simulink model "Quadrotor_Model_PID_Control"  (R2023b)
settings: Solver=VariableStepAuto  StartTime=0.0  StopTime=10.0  RelTol=1e-3
values from neighbouring files (symbols this model uses):
  b = 1.140 * 10^-7    (= 1.14e-07)    [Quadrotor_PID_Parameter_Trial_Updated.m]
  g = 9.82    [Quadrotor_PID_Parameter_Trial_Updated.m]
  I_xx = 4.856 * 10^-3    (= 0.004856)    [Quadrotor_PID_Parameter_Trial_Updated.m]
  I_yy = 4.856 * 10^-3    (= 0.004856)    [Quadrotor_PID_Parameter_Trial_Updated.m]
  I_zz = 8.801 * 10^-3    (= 0.008801)    [Quadrotor_PID_Parameter_Trial_Updated.m]
  k = 2.980*10^-6    (= 2.98e-06)    [Quadrotor_PID_Parameter_Trial_Updated.m]
  Kdx = 1.5    [Quadrotor_PID_Parameter_Trial_Updated.m]
  Kdy = 2.5    [Quadrotor_PID_Parameter_Trial_Updated.m]
  Kdz = 1    [Quadrotor_PID_Parameter_Trial_Updated.m]
  l = 0.225    [Quadrotor_PID_Parameter_Trial_Updated.m]    (also in Reference_Drone_Updated_PID.m = 0.15)
  m = 0.468    [Quadrotor_PID_Parameter_Trial_Updated.m]
libraries: slpidlib x4
settings Model: Creator=jerss  LastModifiedBy=jerss

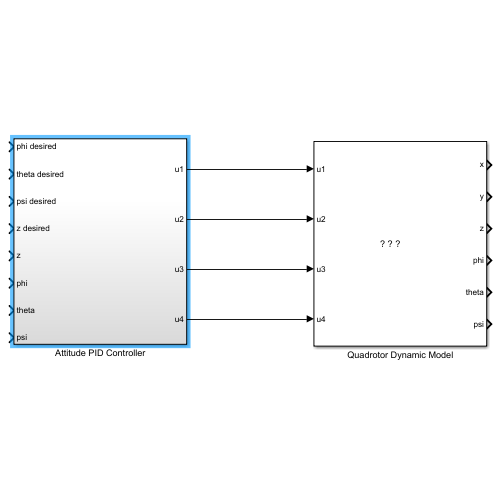
[thumbnail: Simulink's stored preview of the top-level diagram]
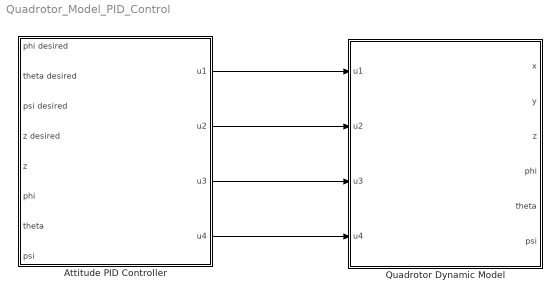
== system Quadrotor_Model_PID_Control ==
  Attitude PID Controller : Subsystem
  Quadrotor Dynamic Model : Subsystem
      mask Display: image('C:\Users\angel\OneDrive - Universidad Politécnica de Yucatán\CIMAT\1st semester\Robotic Systems Modeling and Control\Project\Quadrotor\images\quadrotor.jpg');
  wires:
  Attitude PID Controller/1(u1) -> Quadrotor Dynamic Model/1(u1)
  Attitude PID Controller/2(u2) -> Quadrotor Dynamic Model/2(u2)
  Attitude PID Controller/3(u3) -> Quadrotor Dynamic Model/3(u3)
  Attitude PID Controller/4(u4) -> Quadrotor Dynamic Model/4(u4)

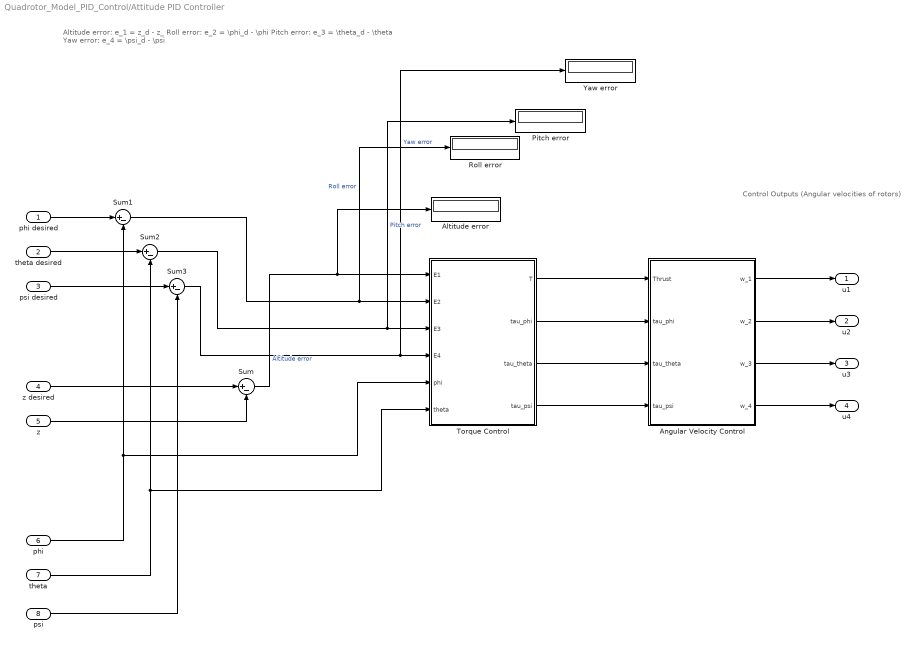
== system Quadrotor_Model_PID_Control/Attitude PID Controller ==
  note: Control Outputs
      | (Angular velocities of rotors)
  note: Altitude error: e_1 = z_d - z_
      | Roll error: e_2 = \phi_d - \phi
      | Pitch error: e_3 = \theta_d - \theta
      | Yaw error: e_4 = \psi_d - \psi
  phi desired : Inport
  theta desired : Inport  Port=2
  psi desired : Inport  Port=3
  z desired : Inport  Port=4
  z : Inport  Port=5
  phi : Inport  Port=6
  theta : Inport  Port=7
  psi : Inport  Port=8
  Altitude error : Display
  Angular Velocity Control : Subsystem
  Pitch error : Display
  Roll error : Display
  Sum{,1..3} (4 alike) : Sum  Inputs=|+-
  Torque Control : Subsystem
  Yaw error : Display
  u1 : Outport
  u2 : Outport  Port=2
  u3 : Outport  Port=3
  u4 : Outport  Port=4
  wires:
  z desired/1 -> Sum/1
  z/1 -> Sum/2
  Sum/1 -> Altitude error/1, Torque Control/1(E1)  "Altitude error"
  phi desired/1 -> Sum1/1
  phi/1 -> Torque Control/5("phi "), Sum1/2
  theta desired/1 -> Sum2/1
  theta/1 -> Sum2/2, Torque Control/6("theta ")
  psi desired/1 -> Sum3/1
  psi/1 -> Sum3/2
  Sum1/1 -> Roll error/1, Torque Control/2(E2)  "Roll error"
  Sum2/1 -> Pitch error/1, Torque Control/3(E3)  "Pitch error"
  Sum3/1 -> Torque Control/4(E4), Yaw error/1  "Yaw error"
  Torque Control/2(tau_phi) -> Angular Velocity Control/2(tau_phi)
  Torque Control/1(T) -> Angular Velocity Control/1(Thrust)
  Torque Control/3(tau_theta) -> Angular Velocity Control/3(tau_theta)
  Torque Control/4(tau_psi) -> Angular Velocity Control/4("tau_psi ")
  Angular Velocity Control/1(w_1) -> u1/1
  Angular Velocity Control/2(w_2) -> u2/1
  Angular Velocity Control/3(w_3) -> u3/1
  Angular Velocity Control/4("w_4 ") -> u4/1

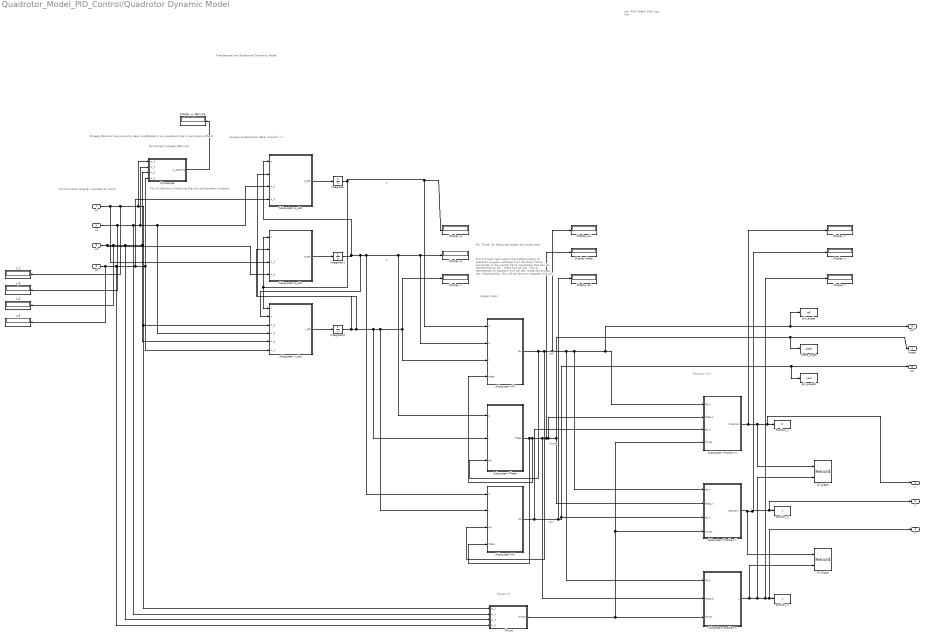
== system Quadrotor_Model_PID_Control/Quadrotor Dynamic Model ==
  note: Phi, Theta, Psi Measured angles dot inside here
  note: This W_Gamma is following the plus configuration currently
  note: Omega_Gamma have currently been unreflected in our equations due to gyroscopic effects
  note: This full block talks about the trabsformation of quadrotor angular velocities from the body frame coordinate to the inertial frame coordinate that can be represented by phi , theta and psi dot - this is represented by equation 6 of phi dot, theta dot and psi dot.
      | Subsequently, this will be done to integrate it to phi, theta and psi.
  note: Angular Accelerations (Body Frame) (\nu)
  note: .
  note: \phi: Roll
      | \theta: Pitch
      | \psi: Yaw
  note: Control Inputs
      | (Angular velocities of rotors)
  note: Positions (\xi)
  note: Angles (\eta)
  note: Gyroscope (\omega_\Gamma)
  note: Thrust (T)
  note: p
  note: q
  note: r
  note: \phi
  note: \theta
  note: \psi
  note: Translational and Rotational Dynamics Model
  u1 : Inport
  u2 : Inport  Port=2
  u3 : Inport  Port=3
  u4 : Inport  Port=4
  Display p : Display
  Display phi : Display
  Display psi : Display
  Display q : Display
  Display r : Display
  Display theta : Display
  Display w_Gamma : Display
  Display x : Display
  Display y : Display
  Display z : Display
  Gyroscope : MATLAB Function  TreatAsAtomicUnit=on
  Integrator : Integrator
  Integrator1 : Integrator
  Integrator2 : Integrator
  Position_x : ToWorkspace  VariableName=X  SampleTime=-1
  Subsystem Phi : Subsystem
  Subsystem Position X : Subsystem
  Subsystem Position Y : Subsystem
  Subsystem Psi : Subsystem
  Subsystem Theta : Subsystem
  Subsystem p_dot : Subsystem
  Subsystem position z : Subsystem
  Subsystem q_dot : Subsystem
  Subsystem r_dot : Subsystem
  Thrust : MATLAB Function  TreatAsAtomicUnit=on
  XZ graph : Record  FileSettingsInternal="{\"entries\":[{\"content\":{\"excelSettings\":{\"content\":{},\"type\":\"Streamout.ExcelSettings\"}},\"type\":\"Streamout.FileSettingStorage\",\"uuid\":\"\"}],\"packageUris\":[\"http:\\/\\/schema.mathworks.com\\/mf0\\/streamout_blocks\\/R2020a\"],\"version\":\"1.0\"}"  Layout=[1 1]  SignalsInternal="{\"entries\":[{\"content\":{\"signals\":[{\"content\":{\"blockPath\":[],\"dimensions\":[1],\"domain\":\"\",\"lineColor\":\"#a2142f\",\"plots\":[1],\"port\":1,\"signalID\":16,\"signalName\":\"Subsystem position x\"},\"type\":\"RecordBlkView.Signal\",\"uuid\":\"\"},{\"content\":{\"blockPath\":[],\"dimensions\":[1],\"domain\":\"\",\"lineColor\":\"#139fff\",\"plots\":[1],\"port\":2,\"signalID\":19,\"signalName\":\"Subsystem position z\"},\"type\":\"RecordBlkView.Signal\",\"uuid\":\"\"}]},\"type\":\"RecordBlkView.InputSignals\",\"uuid\":\"\"}],\"packageUris\":[\"http:\\/\\/schema.mathworks.com\\/mf0\\/streamout_blocks\\/R2020a\"],\"version\":\"1.0\"}"  VisualizationBindings="{\"xyplotplugin\":{\"info\":[{\"series\":[{\"bindingParametersList\":[{\"parameter\":\"X-Axis\",\"signalID\":16,\"signalName\":\"Subsystem position x\"},{\"parameter\":\"Y-Axis\",\"signalID\":19,\"signalName\":\"Subsystem position z\"}],\"seriesID\":56291}],\"subplotID\":1}]}}"  CompatibilityTag=XY  st=-1
  YZ Graph : Record  FileSettingsInternal="{\"entries\":[{\"content\":{\"excelSettings\":{\"content\":{},\"type\":\"Streamout.ExcelSettings\"}},\"type\":\"Streamout.FileSettingStorage\",\"uuid\":\"\"}],\"packageUris\":[\"http:\\/\\/schema.mathworks.com\\/mf0\\/streamout_blocks\\/R2020a\"],\"version\":\"1.0\"}"  Layout=[1 1]  SignalsInternal="{\"entries\":[{\"content\":{\"signals\":[{\"content\":{\"blockPath\":[],\"dimensions\":[1],\"domain\":\"\",\"lineColor\":\"#a2142f\",\"plots\":[1],\"port\":1,\"signalID\":8,\"signalName\":\"Subsystem position y\"},\"type\":\"RecordBlkView.Signal\",\"uuid\":\"\"},{\"content\":{\"blockPath\":[],\"dimensions\":[1],\"domain\":\"\",\"lineColor\":\"#139fff\",\"plots\":[1],\"port\":2,\"signalID\":11,\"signalName\":\"Subsystem position z\"},\"type\":\"RecordBlkView.Signal\",\"uuid\":\"\"}]},\"type\":\"RecordBlkView.InputSignals\",\"uuid\":\"\"}],\"packageUris\":[\"http:\\/\\/schema.mathworks.com\\/mf0\\/streamout_blocks\\/R2020a\"],\"version\":\"1.0\"}"  VisualizationBindings="{\"xyplotplugin\":{\"info\":[{\"series\":[{\"bindingParametersList\":[{\"parameter\":\"X-Axis\",\"signalID\":8,\"signalName\":\"Subsystem position y\"},{\"parameter\":\"Y-Axis\",\"signalID\":11,\"signalName\":\"Subsystem position z\"}],\"seriesID\":24584}],\"subplotID\":1}]}}"  CompatibilityTag=XY  st=-1
  phi_angle : ToWorkspace  VariableName=roll  SampleTime=-1
  phi_angle1 : ToWorkspace  VariableName=yaw  SampleTime=-1
  position_y : ToWorkspace  VariableName=y  SampleTime=-1
  position_z : ToWorkspace  VariableName=z  SampleTime=-1
  theta_angle : ToWorkspace  VariableName=pitch  SampleTime=-1
  u_{1..4} (4 alike) : Display
  x : Outport
  y : Outport  Port=2
  z : Outport  Port=3
  phi : Outport  Port=4
  theta : Outport  Port=5
  psi : Outport  Port=6
  wires:
  u1/1 -> Subsystem q_dot/3(w_1), u_1/1, Gyroscope/1(w_1), Subsystem r_dot/3(w_1), Thrust/1(w_1)
  u2/1 -> Subsystem p_dot/3(w_2), Subsystem r_dot/4(w_2), Gyroscope/2(w_2), Thrust/2(w_2), u_2/1
  u3/1 -> Subsystem q_dot/4(w_3), Gyroscope/3(w_3), Subsystem r_dot/5(w_3), Thrust/3(w_3), u_3/1
  u4/1 -> u_4/1, Gyroscope/4(w_4), Subsystem r_dot/6(w_4), Subsystem p_dot/4(w_4), Thrust/4(w_4)
  Thrust/1(Thrust) -> Subsystem Position X/4(Thrust), Subsystem Position Y/4("Thrust "), Subsystem position z/3(Thrust)
  Subsystem Phi/1("Phi ") -> Subsystem Theta/3("phi "), Subsystem Psi/3(Phi), Display phi/1, Subsystem position z/1("Phi Z "), Subsystem Position Y/1("Phi Y "), phi/1, phi_angle/1, Subsystem Position X/1("Phi X ")
  Subsystem Psi/1(Psi) -> Subsystem Position X/3("Psi X "), Display psi/1, phi_angle1/1, psi/1, Subsystem Position Y/3("Psi Y ")
  Subsystem Position X/1(X Position) -> Display x/1, x/1, Position_x/1, XZ graph/1
  Subsystem position z/1(z) -> YZ Graph/2, XZ graph/2, z/1, position_z/1, Display z/1
  Subsystem Position Y/1("Position Y ") -> y/1, position_y/1, Display y/1, YZ Graph/1
  Gyroscope/1(w_Gamma) -> Display w_Gamma/1
  Subsystem p_dot/1(p_dot) -> Integrator/1
  Subsystem q_dot/1(q_dot) -> Integrator1/1
  Subsystem r_dot/1(r_dot) -> Integrator2/1
  Integrator/1 -> Display p/1, Subsystem Phi/1(p), Subsystem r_dot/1("p "), Subsystem q_dot/1("p ")
  Integrator2/1 -> Subsystem Theta/2(r), Subsystem Psi/2(r), Display r/1, Subsystem Phi/3(r), Subsystem p_dot/2(r), Subsystem q_dot/2(r)
  Integrator1/1 -> Subsystem p_dot/1(q), Subsystem Psi/1(q), Subsystem Theta/1(q), Display q/1, Subsystem Phi/2(q), Subsystem r_dot/2(q)
  Subsystem Theta/1(Theta) -> Subsystem Psi/4(Theta), Subsystem Phi/4(theta), Subsystem position z/2("Theta Z "), Display theta/1, Subsystem Position X/2("Theta X "), theta_angle/1, theta/1, Subsystem Position Y/2("Theta Y ")

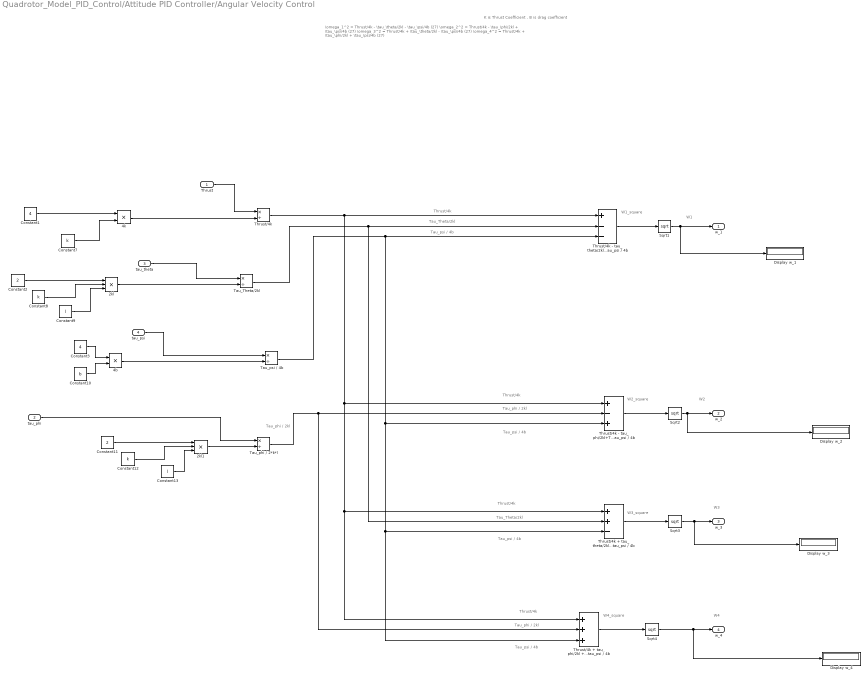
== system Quadrotor_Model_PID_Control/Attitude PID Controller/Angular Velocity Control ==
  note: Tau_psi / 4b
  note: Tau_Theta/2kl
  note: Thrust/4k
  note: W1_square
  note: K is Thrust Coefficient , B is drag coefficient
  note: \omega_1^2 = Thrust/4k - \tau_\theta/2kl - \tau_\psi/4b   (27)
      |
      | \omega_2^2 = Thrust/4k - \tau_\phi/2kl + \tau_\psi/4b   (27)
      |
      | \omega_3^2 = Thrust/4k + \tau_\theta/2kl - \tau_\psi/4b   (27)
      |
      | \omega_4^2 = Thrust/4k + \tau_\phi/2kl + \tau_\psi/4b   (27)
  note: W1
  note: Thrust/4k
  note: Tau_phi / 2kl
  note: Tau_psi / 4b
  note: W2_square
  note: W2
  note: Thrust/4k
  note: W3
  note: W3_square
  note: Tau_Theta/2kl
  note: Tau_psi / 4b
  note: W4_square
  note: W4
  note: Thrust/4k
  note: Tau_phi / 2kl
  note: Tau_phi / 2kl
  note: Tau_psi / 4b
  Thrust : Inport
  tau_phi : Inport  Port=2
  tau_theta : Inport  Port=3
  "tau_psi " : Inport  Port=4
  2kl : Product  Inputs=***
  2kl1 : Product  Inputs=***
  4b : Product  Inputs=**
  4k : Product  Inputs=**
  Constant1 : Constant  Value=4
  Constant10 : Constant  Value=b
  Constant11 : Constant  Value=2
  Constant12 : Constant  Value=k
  Constant13 : Constant  Value=l
  Constant2 : Constant  Value=2
  Constant3 : Constant  Value=4
  Constant7 : Constant  Value=k
  Constant8 : Constant  Value=k
  Constant9 : Constant  Value=l
  Display w_{1..4} (4 alike) : Display
  Sqrt1 : Sqrt
  Sqrt2 : Sqrt  OutputSignalType=real
  Sqrt3 : Sqrt
  Sqrt4 : Sqrt
  Tau_Theta/2kl : Product  Inputs=*/
  Tau_phi / 2*k*l : Product  Inputs=*/
  Tau_psi / 4b : Product  Inputs=*/
  Thrust/4k : Product  Inputs=*/
  Thrust/4k + tau_phi/2kl + tau_psi / 4b : Sum  Inputs=+++
  Thrust/4k + tau_theta/2kl -tau_psi / 4b : Sum  Inputs=++-
  Thrust/4k - tau_phi/2kl+Tau_psi / 4b : Sum  Inputs=+-+
  Thrust/4k - tau_theta/2kl-Tau_psi / 4b : Sum  Inputs=+--
  w_1 : Outport
  w_2 : Outport  Port=2
  w_3 : Outport  Port=3
  "w_4 " : Outport  Port=4
  wires:
  tau_theta/1 -> Tau_Theta/2kl/1
  Sqrt1/1 -> Display w_1/1, w_1/1
  tau_phi/1 -> Tau_phi / 2*k*l/1
  "tau_psi "/1 -> Tau_psi / 4b/1
  Sqrt2/1 -> Display w_2/1, w_2/1
  Thrust/4k - tau_phi/2kl+Tau_psi / 4b/1 -> Sqrt2/1
  Thrust/4k + tau_theta/2kl -tau_psi / 4b/1 -> Sqrt3/1
  Sqrt3/1 -> Display w_3/1, w_3/1
  Thrust/4k + tau_phi/2kl + tau_psi / 4b/1 -> Sqrt4/1
  Sqrt4/1 -> Display w_4/1, "w_4 "/1
  Constant1/1 -> 4k/1
  Constant7/1 -> 4k/2
  Constant8/1 -> 2kl/2
  Constant2/1 -> 2kl/1
  2kl/1 -> Tau_Theta/2kl/2
  Constant9/1 -> 2kl/3
  Constant3/1 -> 4b/1
  Constant10/1 -> 4b/2
  4k/1 -> Thrust/4k/2
  Constant11/1 -> 2kl1/1
  Constant12/1 -> 2kl1/2
  Constant13/1 -> 2kl1/3
  Thrust/1 -> Thrust/4k/1
  4b/1 -> Tau_psi / 4b/2
  2kl1/1 -> Tau_phi / 2*k*l/2
  Thrust/4k/1 -> Thrust/4k + tau_theta/2kl -tau_psi / 4b/1, Thrust/4k + tau_phi/2kl + tau_psi / 4b/1, Thrust/4k - tau_phi/2kl+Tau_psi / 4b/1, Thrust/4k - tau_theta/2kl-Tau_psi / 4b/1
  Tau_Theta/2kl/1 -> Thrust/4k - tau_theta/2kl-Tau_psi / 4b/2, Thrust/4k + tau_theta/2kl -tau_psi / 4b/2
  Thrust/4k - tau_theta/2kl-Tau_psi / 4b/1 -> Sqrt1/1
  Tau_phi / 2*k*l/1 -> Thrust/4k + tau_phi/2kl + tau_psi / 4b/2, Thrust/4k - tau_phi/2kl+Tau_psi / 4b/2
  Tau_psi / 4b/1 -> Thrust/4k - tau_theta/2kl-Tau_psi / 4b/3, Thrust/4k - tau_phi/2kl+Tau_psi / 4b/3, Thrust/4k + tau_phi/2kl + tau_psi / 4b/3, Thrust/4k + tau_theta/2kl -tau_psi / 4b/3

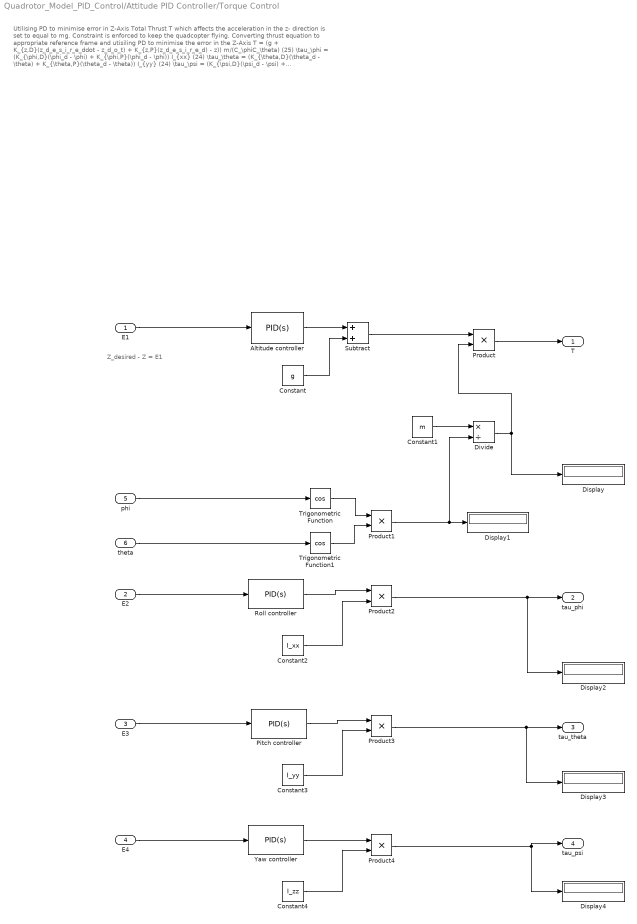
== system Quadrotor_Model_PID_Control/Attitude PID Controller/Torque Control ==
  note: Z_desired - Z = E1
  note: Utilising PD to minimise error in Z-Axis
      | Total Thrust T which affects the acceleration in the z- direction is set to equal to mg.
      | Constraint is enforced to keep the quadcopter flying.
      | Converting thrust equation to appropriate reference frame and utisiling PD to minimise the error in the Z-Axis
      |
      | T = (g + K_{z,D}(z_d_e_s_i_r_e_ddot - z_d_o_t) + K_{z,P}(z_d_e_s_i_r_e_d) - z)) m/(C_\phiC_\theta)     (25)
      |
      | \tau_\phi = (K_{\phi,D}(\phi_d - \phi) + K_{\phi,P}(\phi_d - \phi)) I_{xx}                   (24)
      |
      | \tau_\theta = (K_{\theta,D}(\theta_d - \theta) + K_{\theta,P}(\theta_d - \theta)) I_{yy}                    (24)
      |
      | \tau_\psi = (K_{\psi,D}(\psi_d - \psi) + K_{\psi,P}(\psi_d - \psi)) I_{zz}                (24)
  E1 : Inport
  E2 : Inport  Port=2
  E3 : Inport  Port=3
  E4 : Inport  Port=4
  "phi " : Inport  Port=5
  "theta " : Inport  Port=6
  Altitude controller : slpidlib/PID Controller  Controller=PID  Form=Parallel  TimeDomain=Continuous-time  UseExternalTs=off  SampleTime=-1  IntegratorMethod=Forward Euler  FilterMethod=Forward Euler  ControllerParametersSource=internal  P=57  I=0.001  UseKiTs=off  D=23  N=572.770791824146  UseFilter=on  TunerSelectOption=Transfer Function Based (PID Tuner App)  InitialConditionSource=internal  InitialConditionForIntegrator=0  InitialConditionForFilter=0  DifferentiatorICPrevScaledInput=0  ExternalReset=none  TrackingMode=off  Kt=1  LimitOutput=on  SatLimitsSource=internal  UpperSaturationLimit=5  LowerSaturationLimit=-5  LinearizeAsGain=on  AntiWindupMode=none  Kb=1  LimitIntegrator=off  UpperIntegratorSaturationLimit=inf  LowerIntegratorSaturationLimit=-inf  POutMin=[]  POutMax=[]  IOutMin=[]  IOutMax=[]  DOutMin=[]  DOutMax=[]  NOutMin=[]  NOutMax=[]  SumOutMin=[]  SumOutMax=[]  SaturationOutMin=[]  SaturationOutMax=[]  PParamMin=[]  PParamMax=[]  IParamMin=[]  IParamMax=[]  DParamMin=[]  DParamMax=[]  NParamMin=[]  NParamMax=[]  KbParamMin=[]  KbParamMax=[]  KtParamMin=[]  KtParamMax=[]  KbOutMin=[]  KbOutMax=[]  KtOutMin=[]  KtOutMax=[]  IntegratorOutMin=[]  IntegratorOutMax=[]  FilterOutMin=[]  FilterOutMax=[]  SumI1OutMin=[]  SumI1OutMax=[]  SumI2OutMin=[]  SumI2OutMax=[]  SumI3OutMin=[]  SumI3OutMax=[]  SumI4OutMin=[]  SumI4OutMax=[]  SumDOutMin=[]  SumDOutMax=[]  DifferentiatorOutMin=[]  DifferentiatorOutMax=[]  FilterDiffOutCoefMin=[]  FilterDiffOutCoefMax=[]  ReciprocalOutMin=[]  ReciprocalOutMax=[]  SumDenOutMin=[]  SumDenOutMax=[]  SumNumOutMin=[]  SumNumOutMax=[]  DivideOutMin=[]  DivideOutMax=[]  UdiffTsProdOutMin=[]  UdiffTsProdOutMax=[]  NTsProdOutMin=[]  NTsProdOutMax=[]  UintegralTsProdOutMin=[]  UintegralTsProdOutMax=[]  UngainTsProdOutMin=[]  UngainTsProdOutMax=[]  ClampingZeroOutDataTypeStr=Inherit: Inherit via back propagation  ClampingZeroOutMin=[]  ClampingZeroOutMax=[]  FilterDenConstantOutDataTypeStr=Inherit: Inherit via back propagation  FilterDenConstantOutMin=[]  FilterDenConstantOutMax=[]  PCopyOutDataTypeStr=Inherit: Inherit via back propagation  PCopyOutMin=[]  PCopyOutMax=[]  NCopyOutDataTypeStr=Inherit: Inherit via back propagation  NCopyOutMin=[]  NCopyOutMax=[]  IntegratorContinuousStateAttributes=''  IntegratorStateMustResolveToSignalObject=off  IntegratorRTWStateStorageClass=Auto  FilterContinuousStateAttributes=''  FilterStateMustResolveToSignalObject=off  FilterRTWStateStorageClass=Auto  ParallelPVariant=InternalParameters  IdealPVariant=Disabled  IVariant=InternalParameters  DVariant=InternalParameters  IntegratorVariant=Continuous  SatVariant=Enabled  AWVariant=Passthrough  PCopyVariant=Disabled  TRVariant=Disabled  FdbkBlocksVariant=Forward  IdealPFdbkVariant=Disabled  SatFdbkVariant=Disabled  DerivativeFilterVariant=ContFilter  NVariant=InternalParameters  NCopyVariant=Disabled  FilterICVariant=InternalICsFilter  IntegratorICVariant=InternalICs  ExternalResetVariant=Disabled  TRSumVariant=Passthrough  SumFdbkVariant=Disabled  SumVariant=Sum_PID  TsampFilterVariant=InternalTs  TsampNgainVariant=Passthrough  TsampIntegralVariant=Disabled_SignalSpec  ExternalSaturationOutDataTypeStr=Inherit: Same as second input
  Constant : Constant  Value=g
  Constant1 : Constant  Value=m
  Constant2 : Constant  Value=I_xx
  Constant3 : Constant  Value=I_yy
  Constant4 : Constant  Value=I_zz
  Display{,1..4} (5 alike) : Display
  Divide : Product  Inputs=*/
  Pitch controller : slpidlib/PID Controller  Controller=PID  Form=Parallel  TimeDomain=Continuous-time  UseExternalTs=off  SampleTime=-1  IntegratorMethod=Forward Euler  FilterMethod=Forward Euler  ControllerParametersSource=internal  P=55  I=0.01  UseKiTs=off  D=11  N=1414.64809761679  UseFilter=on  TunerSelectOption=Transfer Function Based (PID Tuner App)  InitialConditionSource=internal  InitialConditionForIntegrator=0  InitialConditionForFilter=0  DifferentiatorICPrevScaledInput=0  ExternalReset=none  TrackingMode=off  Kt=1  LimitOutput=on  SatLimitsSource=internal  UpperSaturationLimit=0.9  LowerSaturationLimit=-0.9  LinearizeAsGain=on  AntiWindupMode=none  Kb=1  LimitIntegrator=off  UpperIntegratorSaturationLimit=inf  LowerIntegratorSaturationLimit=-inf  POutMin=[]  POutMax=[]  IOutMin=[]  IOutMax=[]  DOutMin=[]  DOutMax=[]  NOutMin=[]  NOutMax=[]  SumOutMin=[]  SumOutMax=[]  SaturationOutMin=[]  SaturationOutMax=[]  PParamMin=[]  PParamMax=[]  IParamMin=[]  IParamMax=[]  DParamMin=[]  DParamMax=[]  NParamMin=[]  NParamMax=[]  KbParamMin=[]  KbParamMax=[]  KtParamMin=[]  KtParamMax=[]  KbOutMin=[]  KbOutMax=[]  KtOutMin=[]  KtOutMax=[]  IntegratorOutMin=[]  IntegratorOutMax=[]  FilterOutMin=[]  FilterOutMax=[]  SumI1OutMin=[]  SumI1OutMax=[]  SumI2OutMin=[]  SumI2OutMax=[]  SumI3OutMin=[]  SumI3OutMax=[]  SumI4OutMin=[]  SumI4OutMax=[]  SumDOutMin=[]  SumDOutMax=[]  DifferentiatorOutMin=[]  DifferentiatorOutMax=[]  FilterDiffOutCoefMin=[]  FilterDiffOutCoefMax=[]  ReciprocalOutMin=[]  ReciprocalOutMax=[]  SumDenOutMin=[]  SumDenOutMax=[]  SumNumOutMin=[]  SumNumOutMax=[]  DivideOutMin=[]  DivideOutMax=[]  UdiffTsProdOutMin=[]  UdiffTsProdOutMax=[]  NTsProdOutMin=[]  NTsProdOutMax=[]  UintegralTsProdOutMin=[]  UintegralTsProdOutMax=[]  UngainTsProdOutMin=[]  UngainTsProdOutMax=[]  ClampingZeroOutDataTypeStr=Inherit: Inherit via back propagation  ClampingZeroOutMin=[]  ClampingZeroOutMax=[]  FilterDenConstantOutDataTypeStr=Inherit: Inherit via back propagation  FilterDenConstantOutMin=[]  FilterDenConstantOutMax=[]  PCopyOutDataTypeStr=Inherit: Inherit via back propagation  PCopyOutMin=[]  PCopyOutMax=[]  NCopyOutDataTypeStr=Inherit: Inherit via back propagation  NCopyOutMin=[]  NCopyOutMax=[]  IntegratorContinuousStateAttributes=''  IntegratorStateMustResolveToSignalObject=off  IntegratorRTWStateStorageClass=Auto  FilterContinuousStateAttributes=''  FilterStateMustResolveToSignalObject=off  FilterRTWStateStorageClass=Auto  ParallelPVariant=InternalParameters  IdealPVariant=Disabled  IVariant=InternalParameters  DVariant=InternalParameters  IntegratorVariant=Continuous  SatVariant=Enabled  AWVariant=Passthrough  PCopyVariant=Disabled  TRVariant=Disabled  FdbkBlocksVariant=Forward  IdealPFdbkVariant=Disabled  SatFdbkVariant=Disabled  DerivativeFilterVariant=ContFilter  NVariant=InternalParameters  NCopyVariant=Disabled  FilterICVariant=InternalICsFilter  IntegratorICVariant=InternalICs  ExternalResetVariant=Disabled  TRSumVariant=Passthrough  SumFdbkVariant=Disabled  SumVariant=Sum_PID  TsampFilterVariant=InternalTs  TsampNgainVariant=Passthrough  TsampIntegralVariant=Disabled_SignalSpec  ExternalSaturationOutDataTypeStr=Inherit: Same as second input
  Product{,1..4} (5 alike) : Product
  Roll controller : slpidlib/PID Controller  Controller=PID  Form=Parallel  TimeDomain=Continuous-time  UseExternalTs=off  SampleTime=-1  IntegratorMethod=Forward Euler  FilterMethod=Forward Euler  ControllerParametersSource=internal  P=55  I=0.01  UseKiTs=off  D=14.5  N=1414.64809761679  UseFilter=on  TunerSelectOption=Transfer Function Based (PID Tuner App)  InitialConditionSource=internal  InitialConditionForIntegrator=0  InitialConditionForFilter=0  DifferentiatorICPrevScaledInput=0  ExternalReset=none  TrackingMode=off  Kt=1  LimitOutput=on  SatLimitsSource=internal  UpperSaturationLimit=0.9  LowerSaturationLimit=-0.9  LinearizeAsGain=on  AntiWindupMode=none  Kb=1  LimitIntegrator=off  UpperIntegratorSaturationLimit=inf  LowerIntegratorSaturationLimit=-inf  POutMin=[]  POutMax=[]  IOutMin=[]  IOutMax=[]  DOutMin=[]  DOutMax=[]  NOutMin=[]  NOutMax=[]  SumOutMin=[]  SumOutMax=[]  SaturationOutMin=[]  SaturationOutMax=[]  PParamMin=[]  PParamMax=[]  IParamMin=[]  IParamMax=[]  DParamMin=[]  DParamMax=[]  NParamMin=[]  NParamMax=[]  KbParamMin=[]  KbParamMax=[]  KtParamMin=[]  KtParamMax=[]  KbOutMin=[]  KbOutMax=[]  KtOutMin=[]  KtOutMax=[]  IntegratorOutMin=[]  IntegratorOutMax=[]  FilterOutMin=[]  FilterOutMax=[]  SumI1OutMin=[]  SumI1OutMax=[]  SumI2OutMin=[]  SumI2OutMax=[]  SumI3OutMin=[]  SumI3OutMax=[]  SumI4OutMin=[]  SumI4OutMax=[]  SumDOutMin=[]  SumDOutMax=[]  DifferentiatorOutMin=[]  DifferentiatorOutMax=[]  FilterDiffOutCoefMin=[]  FilterDiffOutCoefMax=[]  ReciprocalOutMin=[]  ReciprocalOutMax=[]  SumDenOutMin=[]  SumDenOutMax=[]  SumNumOutMin=[]  SumNumOutMax=[]  DivideOutMin=[]  DivideOutMax=[]  UdiffTsProdOutMin=[]  UdiffTsProdOutMax=[]  NTsProdOutMin=[]  NTsProdOutMax=[]  UintegralTsProdOutMin=[]  UintegralTsProdOutMax=[]  UngainTsProdOutMin=[]  UngainTsProdOutMax=[]  ClampingZeroOutDataTypeStr=Inherit: Inherit via back propagation  ClampingZeroOutMin=[]  ClampingZeroOutMax=[]  FilterDenConstantOutDataTypeStr=Inherit: Inherit via back propagation  FilterDenConstantOutMin=[]  FilterDenConstantOutMax=[]  PCopyOutDataTypeStr=Inherit: Inherit via back propagation  PCopyOutMin=[]  PCopyOutMax=[]  NCopyOutDataTypeStr=Inherit: Inherit via back propagation  NCopyOutMin=[]  NCopyOutMax=[]  IntegratorContinuousStateAttributes=''  IntegratorStateMustResolveToSignalObject=off  IntegratorRTWStateStorageClass=Auto  FilterContinuousStateAttributes=''  FilterStateMustResolveToSignalObject=off  FilterRTWStateStorageClass=Auto  ParallelPVariant=InternalParameters  IdealPVariant=Disabled  IVariant=InternalParameters  DVariant=InternalParameters  IntegratorVariant=Continuous  SatVariant=Enabled  AWVariant=Passthrough  PCopyVariant=Disabled  TRVariant=Disabled  FdbkBlocksVariant=Forward  IdealPFdbkVariant=Disabled  SatFdbkVariant=Disabled  DerivativeFilterVariant=ContFilter  NVariant=InternalParameters  NCopyVariant=Disabled  FilterICVariant=InternalICsFilter  IntegratorICVariant=InternalICs  ExternalResetVariant=Disabled  TRSumVariant=Passthrough  SumFdbkVariant=Disabled  SumVariant=Sum_PID  TsampFilterVariant=InternalTs  TsampNgainVariant=Passthrough  TsampIntegralVariant=Disabled_SignalSpec  ExternalSaturationOutDataTypeStr=Inherit: Same as second input
  Subtract : Sum
  Trigonometric Function : Trigonometry  Operator=cos
  Trigonometric Function1 : Trigonometry  Operator=cos
  Yaw controller : slpidlib/PID Controller  Controller=PID  Form=Parallel  TimeDomain=Continuous-time  UseExternalTs=off  SampleTime=-1  IntegratorMethod=Forward Euler  FilterMethod=Forward Euler  ControllerParametersSource=internal  P=53  I=0.04  UseKiTs=off  D=26.2  N=95.667343116538  UseFilter=on  TunerSelectOption=Transfer Function Based (PID Tuner App)  InitialConditionSource=internal  InitialConditionForIntegrator=0  InitialConditionForFilter=0  DifferentiatorICPrevScaledInput=0  ExternalReset=none  TrackingMode=off  Kt=1  LimitOutput=on  SatLimitsSource=internal  UpperSaturationLimit=5  LowerSaturationLimit=-5  LinearizeAsGain=on  AntiWindupMode=none  Kb=1  LimitIntegrator=off  UpperIntegratorSaturationLimit=inf  LowerIntegratorSaturationLimit=-inf  POutMin=[]  POutMax=[]  IOutMin=[]  IOutMax=[]  DOutMin=[]  DOutMax=[]  NOutMin=[]  NOutMax=[]  SumOutMin=[]  SumOutMax=[]  SaturationOutMin=[]  SaturationOutMax=[]  PParamMin=[]  PParamMax=[]  IParamMin=[]  IParamMax=[]  DParamMin=[]  DParamMax=[]  NParamMin=[]  NParamMax=[]  KbParamMin=[]  KbParamMax=[]  KtParamMin=[]  KtParamMax=[]  KbOutMin=[]  KbOutMax=[]  KtOutMin=[]  KtOutMax=[]  IntegratorOutMin=[]  IntegratorOutMax=[]  FilterOutMin=[]  FilterOutMax=[]  SumI1OutMin=[]  SumI1OutMax=[]  SumI2OutMin=[]  SumI2OutMax=[]  SumI3OutMin=[]  SumI3OutMax=[]  SumI4OutMin=[]  SumI4OutMax=[]  SumDOutMin=[]  SumDOutMax=[]  DifferentiatorOutMin=[]  DifferentiatorOutMax=[]  FilterDiffOutCoefMin=[]  FilterDiffOutCoefMax=[]  ReciprocalOutMin=[]  ReciprocalOutMax=[]  SumDenOutMin=[]  SumDenOutMax=[]  SumNumOutMin=[]  SumNumOutMax=[]  DivideOutMin=[]  DivideOutMax=[]  UdiffTsProdOutMin=[]  UdiffTsProdOutMax=[]  NTsProdOutMin=[]  NTsProdOutMax=[]  UintegralTsProdOutMin=[]  UintegralTsProdOutMax=[]  UngainTsProdOutMin=[]  UngainTsProdOutMax=[]  ClampingZeroOutDataTypeStr=Inherit: Inherit via back propagation  ClampingZeroOutMin=[]  ClampingZeroOutMax=[]  FilterDenConstantOutDataTypeStr=Inherit: Inherit via back propagation  FilterDenConstantOutMin=[]  FilterDenConstantOutMax=[]  PCopyOutDataTypeStr=Inherit: Inherit via back propagation  PCopyOutMin=[]  PCopyOutMax=[]  NCopyOutDataTypeStr=Inherit: Inherit via back propagation  NCopyOutMin=[]  NCopyOutMax=[]  IntegratorContinuousStateAttributes=''  IntegratorStateMustResolveToSignalObject=off  IntegratorRTWStateStorageClass=Auto  FilterContinuousStateAttributes=''  FilterStateMustResolveToSignalObject=off  FilterRTWStateStorageClass=Auto  ParallelPVariant=InternalParameters  IdealPVariant=Disabled  IVariant=InternalParameters  DVariant=InternalParameters  IntegratorVariant=Continuous  SatVariant=Enabled  AWVariant=Passthrough  PCopyVariant=Disabled  TRVariant=Disabled  FdbkBlocksVariant=Forward  IdealPFdbkVariant=Disabled  SatFdbkVariant=Disabled  DerivativeFilterVariant=ContFilter  NVariant=InternalParameters  NCopyVariant=Disabled  FilterICVariant=InternalICsFilter  IntegratorICVariant=InternalICs  ExternalResetVariant=Disabled  TRSumVariant=Passthrough  SumFdbkVariant=Disabled  SumVariant=Sum_PID  TsampFilterVariant=InternalTs  TsampNgainVariant=Passthrough  TsampIntegralVariant=Disabled_SignalSpec  ExternalSaturationOutDataTypeStr=Inherit: Same as second input
  T : Outport
  tau_phi : Outport  Port=2
  tau_theta : Outport  Port=3
  tau_psi : Outport  Port=4
  wires:
  Constant/1 -> Subtract/2
  E1/1 -> Altitude controller/1
  Altitude controller/1 -> Subtract/1
  Subtract/1 -> Product/1
  Constant1/1 -> Divide/1
  Divide/1 -> Product/2, Display/1
  "phi "/1 -> Trigonometric Function/1
  "theta "/1 -> Trigonometric Function1/1
  Trigonometric Function/1 -> Product1/1
  Trigonometric Function1/1 -> Product1/2
  Product1/1 -> Display1/1, Divide/2
  Product/1 -> T/1
  E2/1 -> Roll controller/1
  Roll controller/1 -> Product2/1
  Constant2/1 -> Product2/2
  Product2/1 -> Display2/1, tau_phi/1
  Constant3/1 -> Product3/2
  Pitch controller/1 -> Product3/1
  Constant4/1 -> Product4/2
  Yaw controller/1 -> Product4/1
  E4/1 -> Yaw controller/1
  E3/1 -> Pitch controller/1
  Product3/1 -> Display3/1, tau_theta/1
  Product4/1 -> tau_psi/1, Display4/1

== system Quadrotor_Model_PID_Control/Quadrotor Dynamic Model/Subsystem Phi ==
  note: Angular Velocity of Phi in the Inertial Frame = Wi
  note: \phi
  note: \phi
  note: .
  note: \phi = p + q(S_\phiT_\theta) + r(C_\phiT_\theta) (6)
  note: .
  note: Display for \phi
  p : Inport
  q : Inport  Port=2
  r : Inport  Port=3
  theta : Inport  Port=4
  "Cos_phi " : Trigonometry  Operator=cos
  Display for q*sin(phi)*tan(Theta) : Display
  Display1 : Display
  Display10 : Display
  Integrator6 : Integrator
  Tan Theta : Trigonometry  Operator=tan
  Tan_Theta : Trigonometry  Operator=tan
  p+ q (sphi ttheta) + r( cphi ttheta) : Sum  Inputs=+++
  q*sin(phi)*tan(Theta) : Product  Inputs=3
  r*cos(phi)*tan(theta) : Product  Inputs=3
  sin(phi) : Trigonometry
  "Phi " : Outport
  wires:
  "Cos_phi "/1 -> r*cos(phi)*tan(theta)/1
  r*cos(phi)*tan(theta)/1 -> Display10/1, p+ q (sphi ttheta) + r( cphi ttheta)/1
  theta/1 -> Tan_Theta/1, Tan Theta/1
  Integrator6/1 -> "Cos_phi "/1, Display1/1, sin(phi)/1, "Phi "/1
  Tan Theta/1 -> r*cos(phi)*tan(theta)/3
  p+ q (sphi ttheta) + r( cphi ttheta)/1 -> Integrator6/1
  q/1 -> q*sin(phi)*tan(Theta)/2
  q*sin(phi)*tan(Theta)/1 -> Display for q*sin(phi)*tan(Theta)/1, p+ q (sphi ttheta) + r( cphi ttheta)/3
  p/1 -> p+ q (sphi ttheta) + r( cphi ttheta)/2
  sin(phi)/1 -> q*sin(phi)*tan(Theta)/1
  Tan_Theta/1 -> q*sin(phi)*tan(Theta)/3
  r/1 -> r*cos(phi)*tan(theta)/2

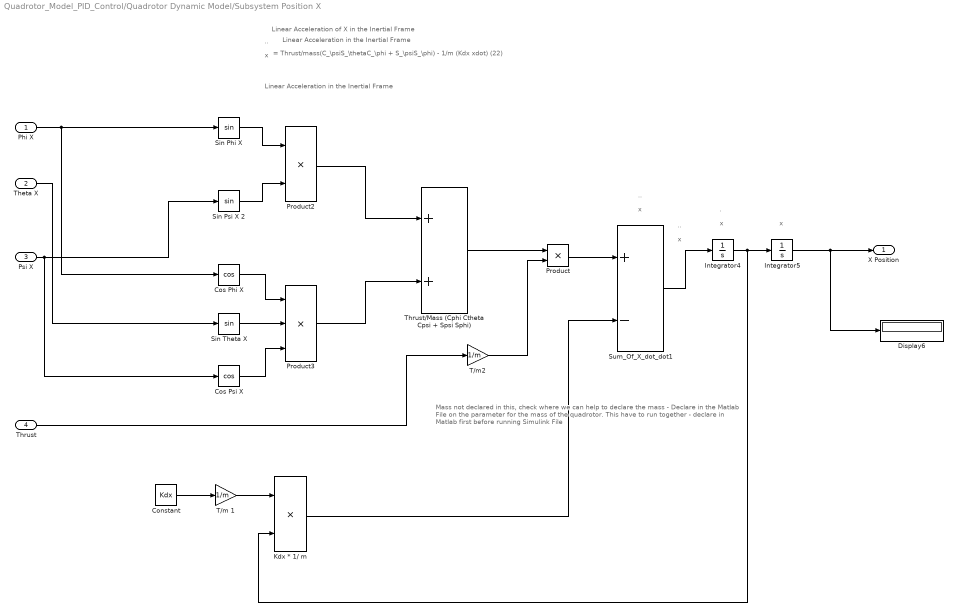
== system Quadrotor_Model_PID_Control/Quadrotor Dynamic Model/Subsystem Position X ==
  note: ..
  note: x
  note: .
  note: x
  note: = Thrust/mass(C_\psiS_\thetaC_\phi + S_\psiS_\phi) - 1/m (Kdx xdot) (22)
  note: ..
  note: x
  note: Linear Acceleration of X in the Inertial Frame
  note: x
  note: Linear Acceleration in the Inertial Frame
  note: Linear Acceleration in the Inertial Frame
  note: Mass not declared in this, check where we can help to declare the mass - Declare in the Matlab File on the parameter for the mass of the quadrotor. This have to run together - declare in Matlab first before running Simulink File
  note: x
  note: ..
  "Phi X " : Inport
  "Theta X " : Inport  Port=2
  "Psi X " : Inport  Port=3
  Thrust : Inport  Port=4
  Constant : Constant  Value=Kdx
  Cos Phi X : Trigonometry  Operator=cos
  Cos Psi X : Trigonometry  Operator=cos
  Display6 : Display
  Integrator4 : Integrator
  Integrator5 : Integrator
  Kdx * 1/ m : Product
  Product : Product
  Product2 : Product
  Product3 : Product  Inputs=3
  Sin Phi X : Trigonometry
  Sin Psi X 2 : Trigonometry
  "Sin Theta X " : Trigonometry
  Sum_Of_X_dot_dot1 : Sum  Inputs=+-
  T/m 1 : Gain  Gain=1/m
  T/m2 : Gain  Gain=1/m
  Thrust/Mass (Cphi Ctheta Cpsi + Spsi Sphi) : Sum
  X Position : Outport
  wires:
  "Phi X "/1 -> Cos Phi X/1, Sin Phi X/1
  "Psi X "/1 -> Sin Psi X 2/1, Cos Psi X/1
  Product2/1 -> Thrust/Mass (Cphi Ctheta Cpsi + Spsi Sphi)/1
  Product3/1 -> Thrust/Mass (Cphi Ctheta Cpsi + Spsi Sphi)/2
  "Theta X "/1 -> "Sin Theta X "/1
  Sin Phi X/1 -> Product2/1
  "Sin Theta X "/1 -> Product3/2
  Sin Psi X 2/1 -> Product2/2
  Cos Psi X/1 -> Product3/3
  Cos Phi X/1 -> Product3/1
  Integrator5/1 -> X Position/1, Display6/1
  T/m2/1 -> Product/2
  Thrust/1 -> T/m2/1
  Thrust/Mass (Cphi Ctheta Cpsi + Spsi Sphi)/1 -> Product/1
  T/m 1/1 -> Kdx * 1/ m/1
  Constant/1 -> T/m 1/1
  Integrator4/1 -> Kdx * 1/ m/2, Integrator5/1
  Product/1 -> Sum_Of_X_dot_dot1/1
  Kdx * 1/ m/1 -> Sum_Of_X_dot_dot1/2
  Sum_Of_X_dot_dot1/1 -> Integrator4/1

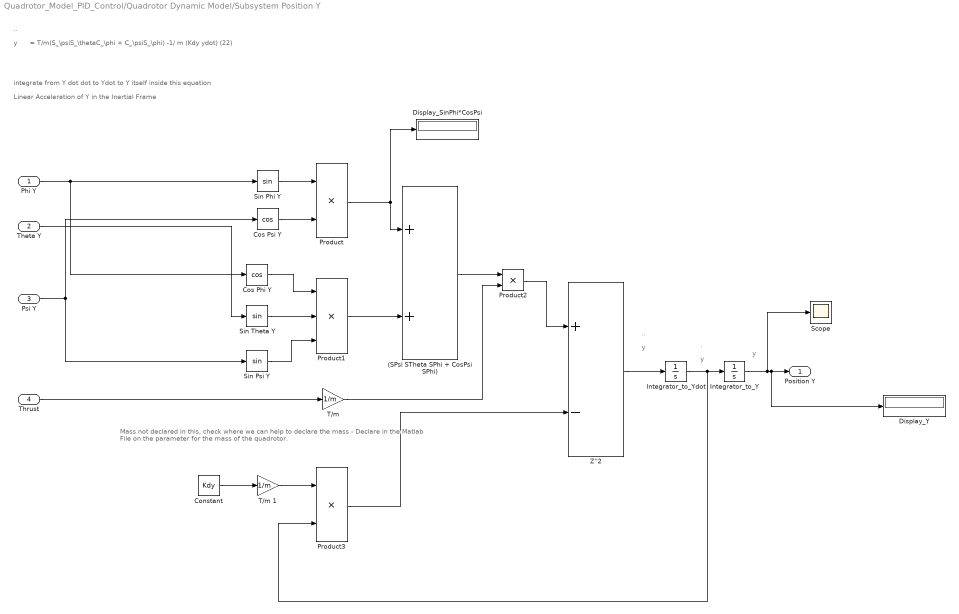
== system Quadrotor_Model_PID_Control/Quadrotor Dynamic Model/Subsystem Position Y ==
  note: Linear Acceleration of Y in the Inertial Frame
  note: integrate from Y dot dot to Ydot to Y itself inside this equation
  note: = T/m(S_\psiS_\thetaC_\phi + C_\psiS_\phi) -1/ m (Kdy ydot) (22)
  note: ..
  note: y
  note: y
  note: .
  note: ..
  note: y
  note: y
  note: Mass not declared in this, check where we can help to declare the mass - Declare in the Matlab File on the parameter for the mass of the quadrotor.
  "Phi Y " : Inport
  "Theta Y " : Inport  Port=2
  "Psi Y " : Inport  Port=3
  "Thrust " : Inport  Port=4
  " (SPsi STheta SPhi + CosPsi SPhi)" : Sum
  Constant : Constant  Value=Kdy
  Cos Phi Y : Trigonometry  Operator=cos
  Cos Psi Y : Trigonometry  Operator=cos
  Display_SinPhi*CosPsi : Display
  Display_Y : Display
  Integrator_to_Y : Integrator
  Integrator_to_Ydot : Integrator
  Product : Product
  Product1 : Product  Inputs=3
  Product2 : Product
  Product3 : Product
  Scope : Scope
  "Sin Phi Y " : Trigonometry
  Sin Psi Y : Trigonometry
  "Sin Theta Y " : Trigonometry
  "T/m " : Gain  Gain=1/m
  T/m 1 : Gain  Gain=1/m
  Z''2 : Sum  Inputs=+-
  "Position Y " : Outport
  wires:
  "Theta Y "/1 -> "Sin Theta Y "/1
  Integrator_to_Y/1 -> Display_Y/1, "Position Y "/1, Scope/1
  "Phi Y "/1 -> "Sin Phi Y "/1, Cos Phi Y/1
  Product/1 -> " (SPsi STheta SPhi + CosPsi SPhi)"/1, Display_SinPhi*CosPsi/1
  Cos Psi Y/1 -> Product/2
  "Psi Y "/1 -> Cos Psi Y/1, Sin Psi Y/1
  Sin Psi Y/1 -> Product1/3
  Product1/1 -> " (SPsi STheta SPhi + CosPsi SPhi)"/2
  Cos Phi Y/1 -> Product1/1
  "Sin Theta Y "/1 -> Product1/2
  "Sin Phi Y "/1 -> Product/1
  " (SPsi STheta SPhi + CosPsi SPhi)"/1 -> Product2/1
  "T/m "/1 -> Product2/2
  "Thrust "/1 -> "T/m "/1
  Integrator_to_Ydot/1 -> Integrator_to_Y/1, Product3/2
  Constant/1 -> T/m 1/1
  T/m 1/1 -> Product3/1
  Product2/1 -> Z''2/1
  Product3/1 -> Z''2/2
  Z''2/1 -> Integrator_to_Ydot/1

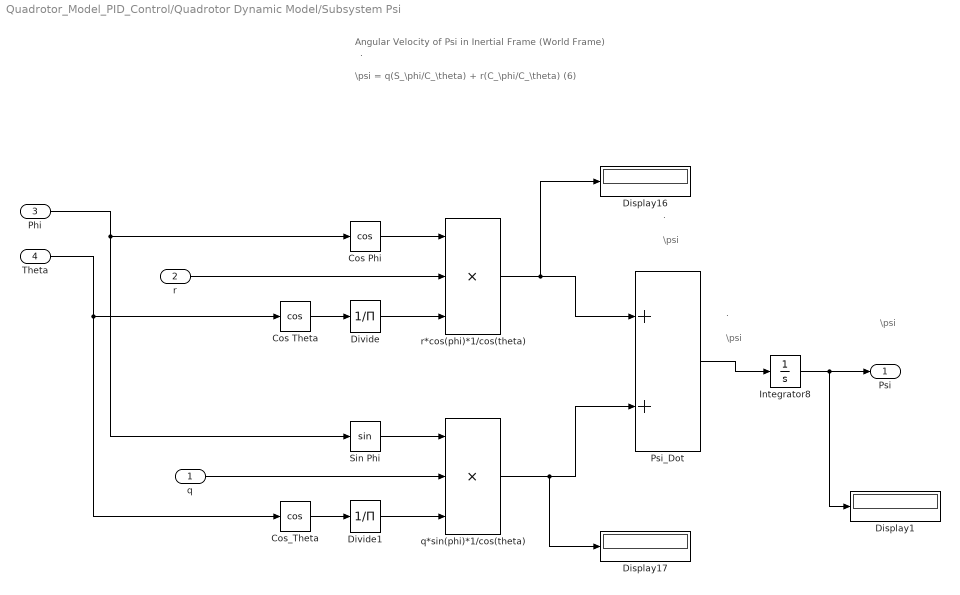
== system Quadrotor_Model_PID_Control/Quadrotor Dynamic Model/Subsystem Psi ==
  note: Angular Velocity of Psi in Inertial Frame (World Frame)
  note: .
  note: \psi
  note: \psi
  note: \psi = q(S_\phi/C_\theta) + r(C_\phi/C_\theta) (6)
  note: .
  note: \psi
  note: .
  q : Inport
  r : Inport  Port=2
  Phi : Inport  Port=3
  Theta : Inport  Port=4
  Cos Phi : Trigonometry  Operator=cos
  Cos Theta : Trigonometry  Operator=cos
  Cos_Theta : Trigonometry  Operator=cos
  Display1 : Display
  Display16 : Display
  Display17 : Display
  Divide : Product  Inputs=/
  Divide1 : Product  Inputs=/
  Integrator8 : Integrator
  Psi_Dot : Sum
  Sin Phi : Trigonometry
  q*sin(phi)*1/cos(theta) : Product  Inputs=3
  r*cos(phi)*1/cos(theta) : Product  Inputs=3
  Psi : Outport
  wires:
  Cos Phi/1 -> r*cos(phi)*1/cos(theta)/1
  Divide1/1 -> q*sin(phi)*1/cos(theta)/3
  Sin Phi/1 -> q*sin(phi)*1/cos(theta)/1
  Cos Theta/1 -> Divide/1
  Divide/1 -> r*cos(phi)*1/cos(theta)/3
  Cos_Theta/1 -> Divide1/1
  r*cos(phi)*1/cos(theta)/1 -> Display16/1, Psi_Dot/1
  Theta/1 -> Cos_Theta/1, Cos Theta/1
  Phi/1 -> Sin Phi/1, Cos Phi/1
  q/1 -> q*sin(phi)*1/cos(theta)/2
  r/1 -> r*cos(phi)*1/cos(theta)/2
  Psi_Dot/1 -> Integrator8/1
  q*sin(phi)*1/cos(theta)/1 -> Psi_Dot/2, Display17/1
  Integrator8/1 -> Display1/1, Psi/1

== system Quadrotor_Model_PID_Control/Quadrotor Dynamic Model/Subsystem Theta ==
  note: Initialise the Pitch Function for parameter initialisation
  note: Angular Velocity of Theta in Inertial Frame (World Frame)
  note: \theta
  note: .
  note: \theta
  note: .
  note: \theta = q(C_\phi) - r(S_\phi) (6)
  note: \theta
  note: .
  q : Inport
  r : Inport  Port=2
  "phi " : Inport  Port=3
  Cos Phi : Trigonometry  Operator=cos
  Display1 : Display
  Display13 : Display
  Display14 : Display
  Integrator_Thetadot to Theta : Integrator
  Sin_Phi : Trigonometry
  Z''4 : Sum  Inputs=-+
  q*cos(phi) : Product
  r*sin(phi) : Product
  Theta : Outport
  wires:
  "phi "/1 -> Cos Phi/1, Sin_Phi/1
  r/1 -> r*sin(phi)/2
  Cos Phi/1 -> q*cos(phi)/1
  q*cos(phi)/1 -> Display14/1, Z''4/2
  Z''4/1 -> Integrator_Thetadot to Theta/1
  Sin_Phi/1 -> r*sin(phi)/1
  r*sin(phi)/1 -> Display13/1, Z''4/1
  q/1 -> q*cos(phi)/2
  Integrator_Thetadot to Theta/1 -> Display1/1, Theta/1

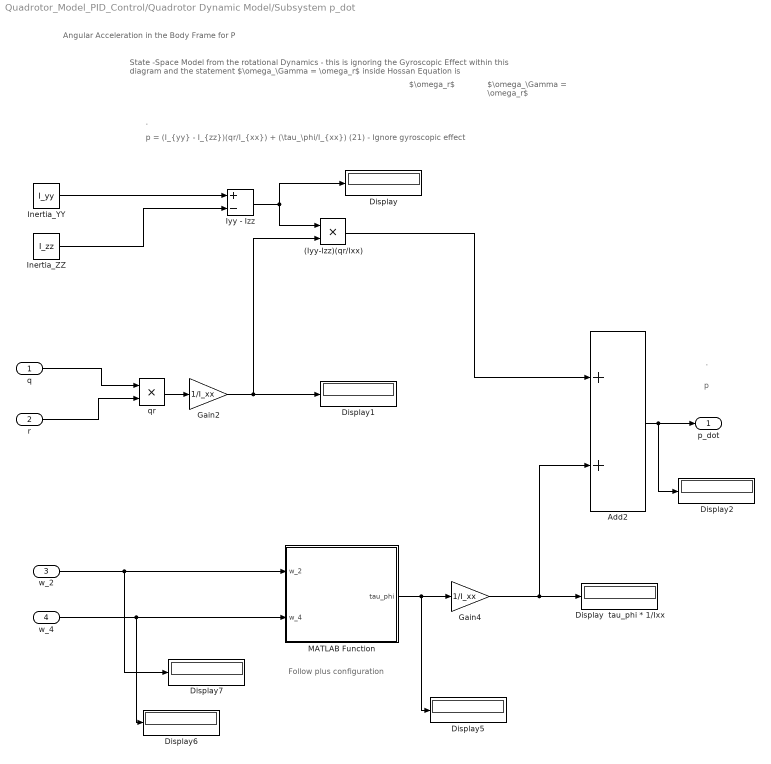
== system Quadrotor_Model_PID_Control/Quadrotor Dynamic Model/Subsystem p_dot ==
  note: .
  note: p
  note: Angular Acceleration in the Body Frame for P
  note: Follow plus configuration
  note: $\omega_r$
  note: $\omega_\Gamma = \omega_r$
  note: State -Space Model from the rotational Dynamics - this is ignoring the Gyroscopic Effect within this diagram and the statement $\omega_\Gamma = \omega_r$ inside Hossan Equation is
  note: p = (I_{yy} - I_{zz})(qr/I_{xx}) + (\tau_\phi/I_{xx}) (21) - Ignore gyroscopic effect
  note: .
  q : Inport
  r : Inport  Port=2
  w_2 : Inport  Port=3
  w_4 : Inport  Port=4
  (Iyy-Izz)(qr/Ixx) : Product
  Add2 : Sum
  Display{,1..2,5..7} (6 alike) : Display
  Display  tau_phi * 1/Ixx : Display
  Gain2 : Gain  Gain=1/I_xx
  Gain4 : Gain  Gain=1/I_xx
  Inertia_YY : Constant  Value=I_yy
  Inertia_ZZ : Constant  Value=I_zz
  Iyy - Izz : Sum  Inputs=+-
  MATLAB Function : MATLAB Function  TreatAsAtomicUnit=on
  qr : Product
  p_dot : Outport
  wires:
  Inertia_YY/1 -> Iyy - Izz/1
  Inertia_ZZ/1 -> Iyy - Izz/2
  Iyy - Izz/1 -> (Iyy-Izz)(qr/Ixx)/1, Display/1
  Add2/1 -> p_dot/1, Display2/1
  q/1 -> qr/1
  MATLAB Function/1(tau_phi) -> Display5/1, Gain4/1
  w_2/1 -> MATLAB Function/1(w_2), Display7/1
  w_4/1 -> Display6/1, MATLAB Function/2(w_4)
  Gain4/1 -> Display  tau_phi * 1/Ixx/1, Add2/2
  r/1 -> qr/2
  qr/1 -> Gain2/1
  Gain2/1 -> (Iyy-Izz)(qr/Ixx)/2, Display1/1
  (Iyy-Izz)(qr/Ixx)/1 -> Add2/1

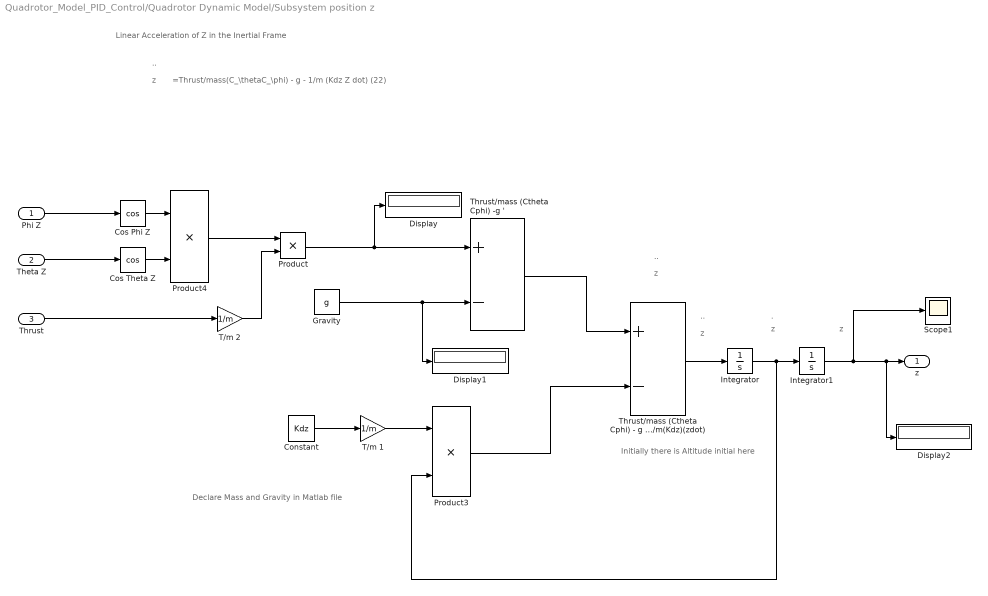
== system Quadrotor_Model_PID_Control/Quadrotor Dynamic Model/Subsystem position z ==
  note: Initially there is Altitude initial here
  note: Linear Acceleration of Z in the Inertial Frame
  note: Declare Mass and Gravity in Matlab file
  note: z
  note: ..
  note: .
  note: z
  note: =Thrust/mass(C_\thetaC_\phi) - g - 1/m (Kdz Z dot) (22)
  note: ..
  note: z
  note: z
  note: ..
  note: z
  "Phi Z " : Inport
  "Theta Z " : Inport  Port=2
  Thrust : Inport  Port=3
  Constant : Constant  Value=Kdz
  Cos Phi Z : Trigonometry  Operator=cos
  Cos Theta Z : Trigonometry  Operator=cos
  Display : Display
  Display1 : Display
  Display2 : Display
  Gravity : Constant  Value=g
  Integrator : Integrator
  Integrator1 : Integrator
  Product : Product
  Product3 : Product
  Product4 : Product
  Scope1 : Scope
  T/m 1 : Gain  Gain=1/m
  T/m 2 : Gain  Gain=1/m
  Thrust/mass (Ctheta Cphi) - g + - 1/m(Kdz)(zdot) : Sum  Inputs=+-
  Thrust/mass (Ctheta Cphi) -g ' : Sum  Inputs=+-
  z : Outport
  wires:
  "Phi Z "/1 -> Cos Phi Z/1
  Gravity/1 -> Display1/1, Thrust/mass (Ctheta Cphi) -g '/2
  Integrator1/1 -> z/1, Display2/1, Scope1/1
  "Theta Z "/1 -> Cos Theta Z/1
  Integrator/1 -> Product3/2, Integrator1/1
  Cos Theta Z/1 -> Product4/2
  Cos Phi Z/1 -> Product4/1
  Thrust/1 -> T/m 2/1
  Product4/1 -> Product/1
  Product/1 -> Display/1, Thrust/mass (Ctheta Cphi) -g '/1
  T/m 2/1 -> Product/2
  T/m 1/1 -> Product3/1
  Constant/1 -> T/m 1/1
  Thrust/mass (Ctheta Cphi) -g '/1 -> Thrust/mass (Ctheta Cphi) - g + - 1/m(Kdz)(zdot)/1
  Product3/1 -> Thrust/mass (Ctheta Cphi) - g + - 1/m(Kdz)(zdot)/2
  Thrust/mass (Ctheta Cphi) - g + - 1/m(Kdz)(zdot)/1 -> Integrator/1

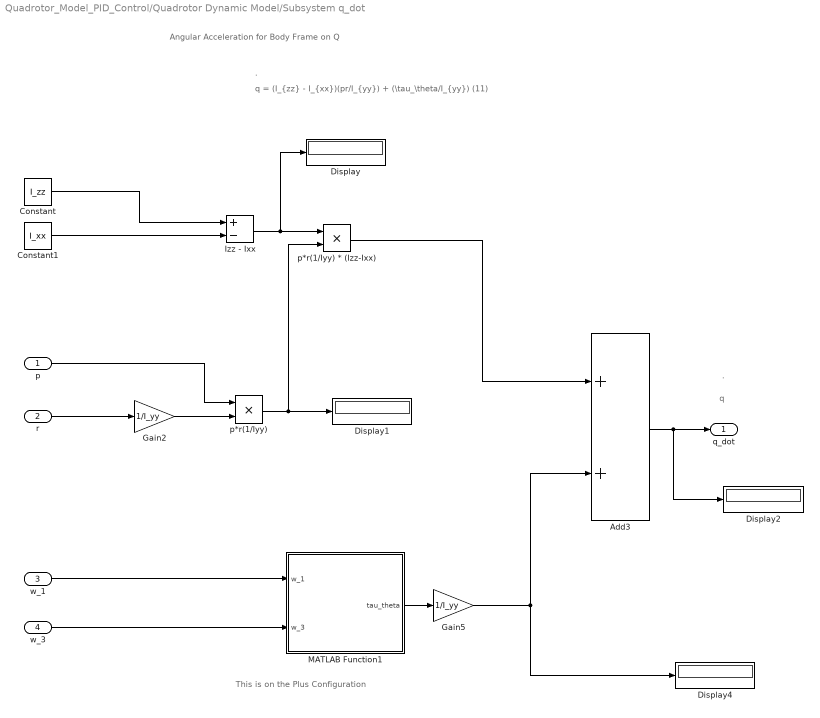
== system Quadrotor_Model_PID_Control/Quadrotor Dynamic Model/Subsystem q_dot ==
  note: .
  note: q
  note: Angular Acceleration for Body Frame on Q
  note: This is on the Plus Configuration
  note: q = (I_{zz} - I_{xx})(pr/I_{yy}) + (\tau_\theta/I_{yy}) (11)
  note: .
  "p " : Inport
  r : Inport  Port=2
  w_1 : Inport  Port=3
  w_3 : Inport  Port=4
  Add3 : Sum
  Constant : Constant  Value=I_zz
  Constant1 : Constant  Value=I_xx
  Display{,1..2,4} (4 alike) : Display
  Gain2 : Gain  Gain=1/I_yy
  Gain5 : Gain  Gain=1/I_yy
  Izz - Ixx : Sum  Inputs=+-
  MATLAB Function1 : MATLAB Function  TreatAsAtomicUnit=on
  p*r(1/Iyy) : Product
  p*r(1/Iyy) * (Izz-Ixx) : Product
  q_dot : Outport
  wires:
  Constant/1 -> Izz - Ixx/1
  Constant1/1 -> Izz - Ixx/2
  Izz - Ixx/1 -> Display/1, p*r(1/Iyy) * (Izz-Ixx)/1
  p*r(1/Iyy)/1 -> p*r(1/Iyy) * (Izz-Ixx)/2, Display1/1
  r/1 -> Gain2/1
  Gain2/1 -> p*r(1/Iyy)/2
  "p "/1 -> p*r(1/Iyy)/1
  w_3/1 -> MATLAB Function1/2(w_3)
  MATLAB Function1/1(tau_theta) -> Gain5/1
  w_1/1 -> MATLAB Function1/1(w_1)
  Add3/1 -> q_dot/1, Display2/1
  Gain5/1 -> Display4/1, Add3/2
  p*r(1/Iyy) * (Izz-Ixx)/1 -> Add3/1

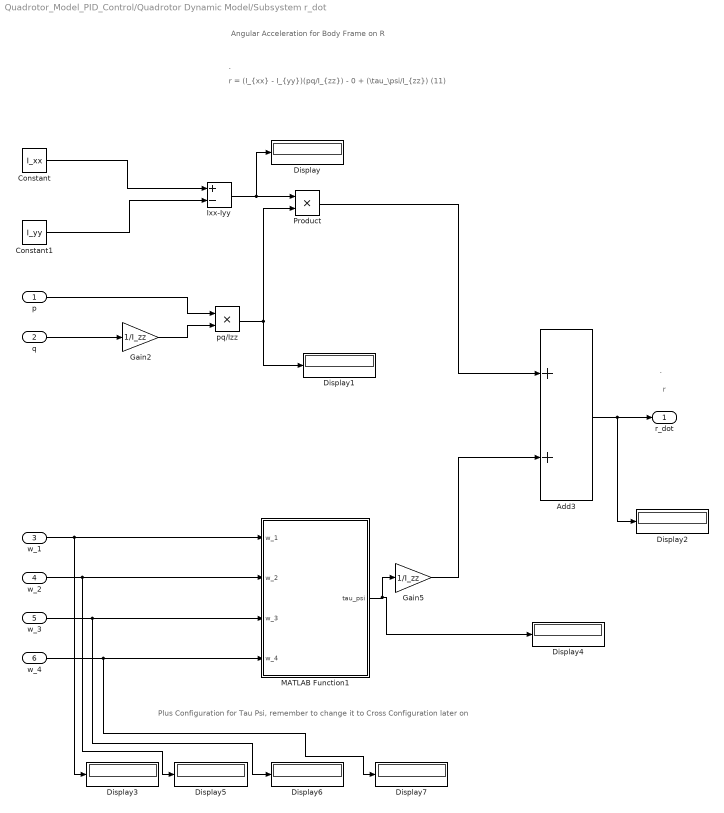
== system Quadrotor_Model_PID_Control/Quadrotor Dynamic Model/Subsystem r_dot ==
  note: r
  note: Plus Configuration for Tau Psi, remember to change it to Cross Configuration later on
  note: Angular Acceleration for Body Frame on R
  note: r = (I_{xx} - I_{yy})(pq/I_{zz}) - 0 + (\tau_\psi/I_{zz}) (11)
  note: .
  note: .
  "p " : Inport
  q : Inport  Port=2
  w_1 : Inport  Port=3
  w_2 : Inport  Port=4
  w_3 : Inport  Port=5
  w_4 : Inport  Port=6
  Add3 : Sum
  Constant : Constant  Value=I_xx
  Constant1 : Constant  Value=I_yy
  Display{,1..7} (8 alike) : Display
  Gain2 : Gain  Gain=1/I_zz
  Gain5 : Gain  Gain=1/I_zz
  Ixx-Iyy : Sum  Inputs=+-
  MATLAB Function1 : MATLAB Function  TreatAsAtomicUnit=on
  Product : Product
  pq/Izz : Product
  r_dot : Outport
  wires:
  Constant/1 -> Ixx-Iyy/1
  Constant1/1 -> Ixx-Iyy/2
  Ixx-Iyy/1 -> Display/1, Product/1
  pq/Izz/1 -> Display1/1, Product/2
  Add3/1 -> Display2/1, r_dot/1
  "p "/1 -> pq/Izz/1
  Gain2/1 -> pq/Izz/2
  q/1 -> Gain2/1
  MATLAB Function1/1(tau_psi) -> Display4/1, Gain5/1
  w_1/1 -> MATLAB Function1/1(w_1), Display3/1
  w_2/1 -> MATLAB Function1/2(w_2), Display5/1
  w_4/1 -> MATLAB Function1/4(w_4), Display7/1
  Gain5/1 -> Add3/2
  w_3/1 -> MATLAB Function1/3(w_3), Display6/1
  Product/1 -> Add3/1

== matlab function Quadrotor_Model_PID_Control/Quadrotor Dynamic Model/Subsystem r_dot/MATLAB Function1 ==
  data: w_1 input; w_2 input; w_3 input; tau_psi output; w_4 input
function tau_psi = fcn(w_1, w_2, w_3, w_4)
k = 2.980e-6; % Thrust factor of rotor (depends on density
              % geometry, etc) 
l = 0.225; % Linear distance from the centre of the rotor
           % to the centre of gravity    
b = 1.140e-7; % Drag constant
Im = 3.357e-5; % Inertia moment of the rotor
tau_psi = b*(-w_1^2 + w_2^2 - w_3^2 + w_4^2); %Plus Configuration
% tau_psi = (b * w_1^2 + Im) - (b * w_2^2 + Im) + (b * w_3^2 + Im) - (b * w_4^2 + Im);

== matlab function Quadrotor_Model_PID_Control/Quadrotor Dynamic Model/Subsystem p_dot/MATLAB Function ==
  data: w_2 input; w_4 input; tau_phi output
function tau_phi = fcn(w_2, w_4)
k = 2.980e-6; % Thrust factor of rotor (depends on density
              % geometry, etc) 
l = 0.225; % Linear distance from the centre of the rotor
           % to the centre of gravity          
tau_phi = l * k * (-w_2^2 + w_4^2);

%Eqn 13

== matlab function Quadrotor_Model_PID_Control/Quadrotor Dynamic Model/Subsystem q_dot/MATLAB Function1 ==
  data: w_1 input; w_3 input; tau_theta output
function tau_theta = fcn(w_1, w_3)
k = 2.980e-6; % Thrust factor of rotor (depends on density
              % geometry, etc) 
l = 0.225; % Linear distance from the centre of the rotor
           % to the centre of gravity          
tau_theta = l * k * (-w_1^2 + w_3^2);

== matlab function Quadrotor_Model_PID_Control/Quadrotor Dynamic Model/Thrust ==
  data: w_1 input; Thrust output; w_2 input; w_3 input; w_4 input
function Thrust = fcn(w_1, w_2, w_3, w_4)
k = 2.980e-6; % Thrust factor of rotor (depends on density)
Thrust = k * (w_1^2 + w_2^2 + w_3^2 + w_4^2);

== matlab function Quadrotor_Model_PID_Control/Quadrotor Dynamic Model/Gyroscope ==
  data: w_1 input; w_2 input; w_3 input; w_Gamma output; w_4 input
function w_Gamma = fcn(w_1, w_2, w_3, w_4)
    
w_Gamma = w_1 - w_2 + w_3 - w_4;
